simulink model "team_project_state_and_cds_adj_integration"  (R2023b)
settings: Solver=FixedStepAuto  StartTime=0.0  StopTime=inf  FixedStep=0.01  RelTol=1e-3  EnableMultiTasking=on
InitFcn:
  | params
  | pin_params
undefined symbols (not defined in the file or in its folder): b, den_Gd, encoder_scale, f, J, Kb, KD, Kf, KI, Km, KP, l, L, num_Gd, r, R, Vlim
libraries: arduinolib x17, arduinosensorlib x6, simulink x2
settings Model: SimulationMode=external  ExtModeTrigDuration=2  Creator=권주성  LastModifiedBy=SJ
settings SolverCC: AutoInsertRateTranBlk=on
settings OptimizationCC: EnhancedBackFolding=on  PassReuseOutputArgsAs=Individual arguments  ZeroExternalMemoryAtStartup=off  ZeroInternalMemoryAtStartup=off  MaxStackSize=64  OptimizeBlockOrder=speed  DifferentSizesBufferReuse=on  OptimizationCustomize=off  EfficientTunableParamExpr=on
settings DebuggingCC: ParameterPrecisionLossMsg=none  ParameterTunabilityLossMsg=error
settings HardwareCC: ProdBitPerInt=16  ProdBitPerPointer=16  ProdBitPerSizeT=16  ProdBitPerPtrDiffT=16  ProdLargestAtomicFloat=None  ProdWordSize=8  ProdHWDeviceType=Atmel->AVR
settings SFSimCC: MATLABDynamicMemAlloc=off
settings RTWCC: Description=Embedded Coder  SystemTargetFile=ert.tlc  HardwareBoard=Arduino Mega 2560  TemplateMakefile=ert_default_tmf  Toolchain=Arduino AVR  BuildConfiguration=Faster Runs
settings CodeAppCC: ForceParamTrailComments=on  IgnoreCustomStorageClasses=off  OperatorAnnotations=on  SimulinkDataObjDesc=on  SFDataObjDesc=on  InsertBlockDesc=on
settings ERTTargetCC: SupportContinuousTime=on  SupportVariableSizeSignals=on  ExtMode=on  ExtModeTransport=3  ExtModeStaticAlloc=on  ExtModeAutomaticAllocSize=off  ExtModeStaticAllocSize=2048  ExtModeMexFile=ext_xcp  ExtModeMexArgs=1 3 921600  ExtModeIntrfLevel=Level2 - Open

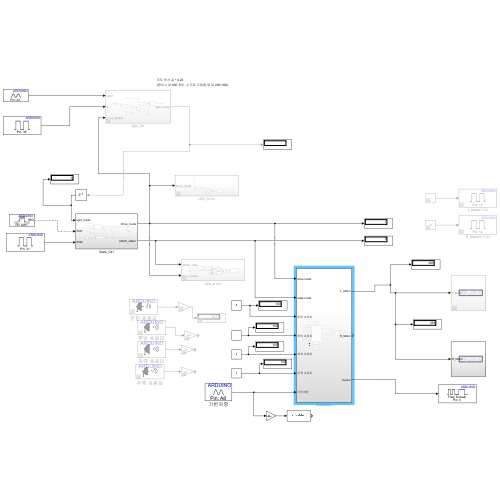
[thumbnail: Simulink's stored preview of the top-level diagram]
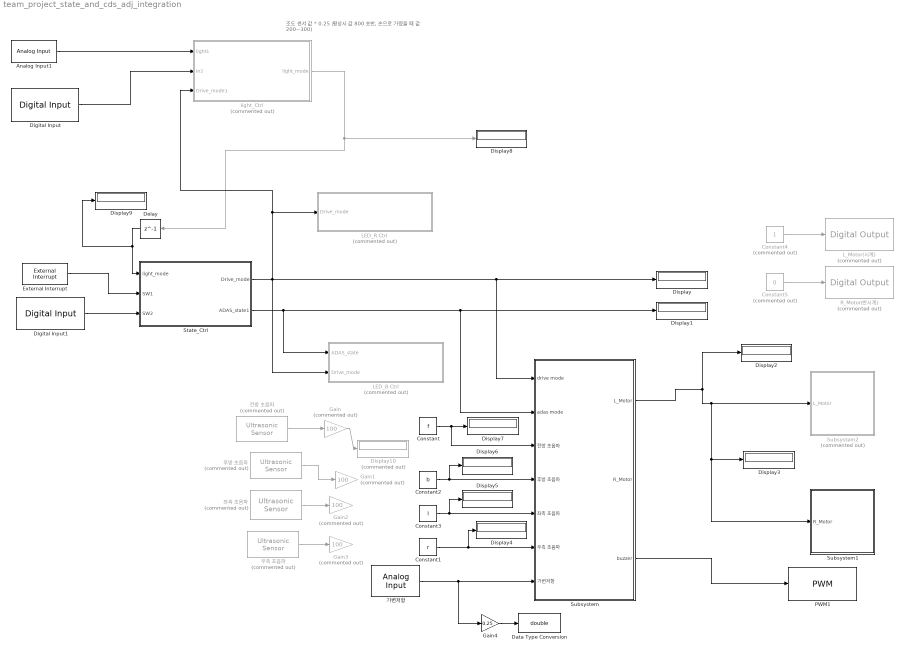
== system team_project_state_and_cds_adj_integration ==
  note: 조도 센서 값 * 0.25
      | (평상시 값 800 초반, 손으로 가렸을 때 값 200~300)
  Analog Input1 : arduinolib/Analog Input  pinNumber=BS  ReadResultsOnly=off  ConversionTriggerSource=Software  ExternalTriggerType=uint32( 0 )  OutputDataType=uint16  EnableConversionCompleteNotify=off  EnableOuputStatus=off  SampleTime=-1  blockPlatform=arduino
  Constant : Constant  Value=f
  Constant1 : Constant  Value=r
  Constant2 : Constant  Value=b
  Constant3 : Constant  Value=l
  Constant4 : Constant  Commented=on
  Constant5 : Constant  Commented=on  Value=0
  Data Type Conversion : DataTypeConversion  OutDataTypeStr=double  SaturateOnIntegerOverflow=off  RndMeth=Floor
  Delay : Delay  DelayLength=1
  Digital Input : arduinolib/Digital Input  pinNumber=SW3  mode=Default  Direction=input  SampleTime=0.1  blockPlatform=arduino
  Digital Input1 : arduinolib/Digital Input  pinNumber=SW2  mode=Default  Direction=input  SampleTime=0.1  blockPlatform=arduino
  Display{,1..9} (10 alike) : Display
  Display10 : Display  Commented=on
  External Interrupt : arduinolib/External Interrupt  Pin=SW1  PullUp=off  Mode=RISING  InterruptSimulationInput=off
  Gain{,1..3} (4 alike) : Gain  Commented=on  Gain=100
  Gain4 : Gain  Gain=0.25
  LED_B Ctrl : Subsystem  Commented=on
  LED_R Ctrl : Subsystem  Commented=on
  L_Motor(시계) : arduinolib/Digital Output  Commented=on  pinNumber=Motor_L_Direction  Direction=output  blockPlatform=arduino
  PWM1 : arduinolib/PWM  pinNumber=Buzzer  frequencyType=Default  desiredFrequency=490.2  achievableFrequency=490.2
  R_Motor(반시계) : arduinolib/Digital Output  Commented=on  pinNumber=Motor_R_Direction  Direction=output  blockPlatform=arduino
  State_Ctrl : Subsystem
  Subsystem : Subsystem
  Subsystem1 : Subsystem
  Subsystem2 : Subsystem  Commented=on
  light_Ctrl : Subsystem  Commented=on
  가변저항 : arduinolib/Analog Input  pinNumber=VR  ReadResultsOnly=off  ConversionTriggerSource=Software  ExternalTriggerType=uint32( 0 )  OutputDataType=uint16  EnableConversionCompleteNotify=off  EnableOuputStatus=off  SampleTime=-1  blockPlatform=arduino
  우측 초음파 : arduinosensorlib/Ultrasonic Sensor  Commented=on  NumSignalPins=2  TrigPin=R_Triger  EchoPin=R_Echo  SignalPin=3  SampleTime_=0.1  blockPlatform=ARDUINO
  전방 초음파 : arduinosensorlib/Ultrasonic Sensor  Commented=on  NumSignalPins=2  TrigPin=F_Triger  EchoPin=F_Echo  SignalPin=3  SampleTime_=0.1  blockPlatform=ARDUINO
  좌측 초음파 : arduinosensorlib/Ultrasonic Sensor  Commented=on  NumSignalPins=2  TrigPin=L_Triger  EchoPin=L_Echo  SignalPin=3  SampleTime_=0.1  blockPlatform=ARDUINO
  후방 초음파 : arduinosensorlib/Ultrasonic Sensor  Commented=on  NumSignalPins=2  TrigPin=B_Triger  EchoPin=B_Echo  SignalPin=3  SampleTime_=0.1  blockPlatform=ARDUINO
  wires:
  light_Ctrl/1(light_mode) -> Display8/1, Delay/1
  Analog Input1/1 -> light_Ctrl/1(light1)
  Delay/1 -> Display9/1, State_Ctrl/1(light_mode)
  State_Ctrl/2(ADAS_state1) -> LED_B Ctrl/1(ADAS_state), Subsystem/2(adas mode), Display1/1
  External Interrupt/1 -> State_Ctrl/2(SW1)
  State_Ctrl/1(Drive_mode) -> Subsystem/1(drive mode), Display/1, light_Ctrl/3(Drive_mode1), LED_R Ctrl/1(Drive_mode), LED_B Ctrl/2(Drive_mode)
  가변저항/1 -> Gain4/1, Subsystem/7(가변저항)
  Subsystem/3(buzzer) -> PWM1/1
  Constant3/1 -> Display5/1, Subsystem/5(좌측 초음파)
  Constant2/1 -> Display6/1, Subsystem/4(후방 초음파)
  좌측 초음파/1 -> Gain2/1
  전방 초음파/1 -> Gain/1
  Constant/1 -> Subsystem/3(전방 초음파), Display7/1
  우측 초음파/1 -> Gain3/1
  Constant1/1 -> Display4/1, Subsystem/6(우측 초음파)
  Subsystem/1(L_Motor) -> Display3/1, Subsystem1/1(R_Motor), Subsystem2/1(L_Motor), Display2/1
  후방 초음파/1 -> Gain1/1
  Digital Input1/1 -> State_Ctrl/3(SW2)
  Digital Input/1 -> light_Ctrl/2(In2)
  Constant4/1 -> L_Motor(시계)/1
  Constant5/1 -> R_Motor(반시계)/1
  Gain/1 -> Display10/1
  Gain4/1 -> Data Type Conversion/1

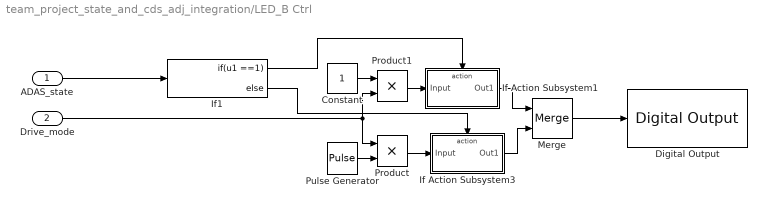
== system team_project_state_and_cds_adj_integration/LED_B Ctrl ==
  ADAS_state : Inport
  Drive_mode : Inport  Port=2
  Constant : Constant
  Digital Output : arduinolib/Digital Output  pinNumber=LED1_B  Direction=output  blockPlatform=arduino
  If Action Subsystem1 : Subsystem  TreatAsAtomicUnit=on
  If Action Subsystem3 : Subsystem  TreatAsAtomicUnit=on
  If1 : If  IfExpression=u1 ==1
  Merge : Merge
  Product : Product
  Product1 : Product
  Pulse Generator : DiscretePulseGenerator  PulseType=Time based  PulseWidth=50
  wires:
  If1/2 -> If Action Subsystem3/Action
  If Action Subsystem1/1(Out1) -> Merge/1
  ADAS_state/1 -> If1/1
  If1/1 -> If Action Subsystem1/Action
  Merge/1 -> Digital Output/1
  If Action Subsystem3/1(Out1) -> Merge/2
  Drive_mode/1 -> Product/1, Product1/2
  Pulse Generator/1 -> Product/2
  Constant/1 -> Product1/1
  Product1/1 -> If Action Subsystem1/1(Input)
  Product/1 -> If Action Subsystem3/1(Input)

== system team_project_state_and_cds_adj_integration/LED_R Ctrl ==
  Drive_mode : Inport
  Digital Output : arduinolib/Digital Output  pinNumber=LED1_R  Direction=output  blockPlatform=arduino
  If Action Subsystem1 : Subsystem  TreatAsAtomicUnit=on
  If Action Subsystem3 : Subsystem  TreatAsAtomicUnit=on
  If1 : If  IfExpression=u1 ==1
  Merge : Merge
  wires:
  If1/2 -> If Action Subsystem3/Action
  If Action Subsystem1/1(Out1) -> Merge/1
  Drive_mode/1 -> If1/1
  If1/1 -> If Action Subsystem1/Action
  Merge/1 -> Digital Output/1
  If Action Subsystem3/1(Out1) -> Merge/2

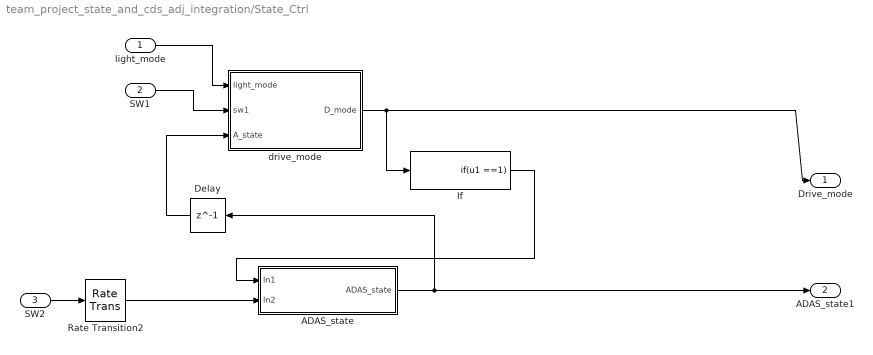
== system team_project_state_and_cds_adj_integration/State_Ctrl ==
  light_mode : Inport
  SW1 : Inport  Port=2
  SW2 : Inport  Port=3
  ADAS_state : Subsystem
  Delay : Delay  DelayLength=1
  If : If  IfExpression=u1 ==1  ShowElse=off
  Rate Transition2 : RateTransition  Integrity=off  OutPortSampleTime=0.2
  drive_mode : Subsystem
  Drive_mode : Outport
  ADAS_state1 : Outport  Port=2
  wires:
  If/1 -> ADAS_state/1(In1)
  drive_mode/1(D_mode) -> If/1, Drive_mode/1
  ADAS_state/1(ADAS_state) -> Delay/1, ADAS_state1/1
  SW1/1 -> drive_mode/2(sw1)
  Delay/1 -> drive_mode/3(A_state)
  light_mode/1 -> drive_mode/1(light_mode)
  SW2/1 -> Rate Transition2/1
  Rate Transition2/1 -> ADAS_state/2(In2)

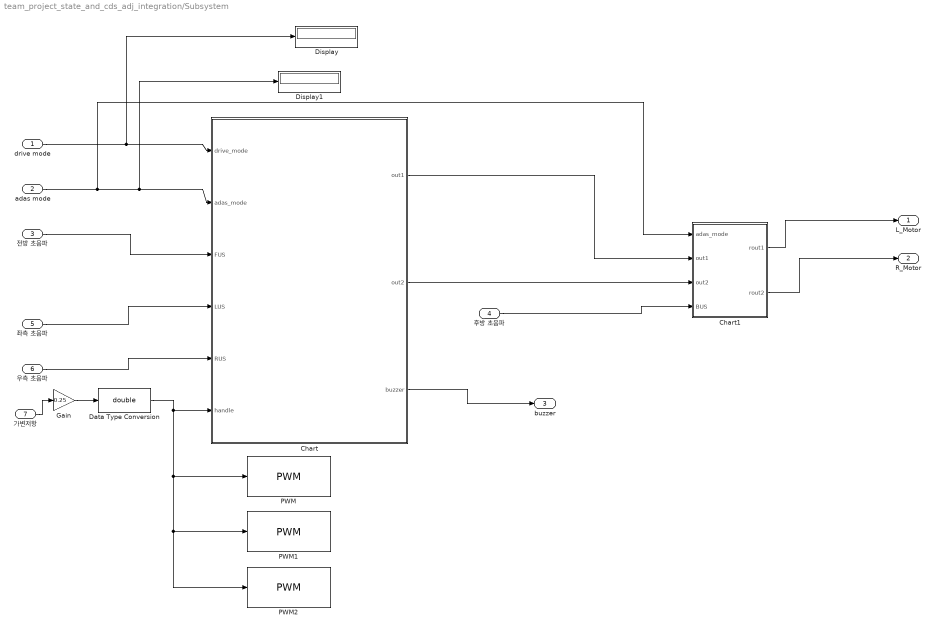
== system team_project_state_and_cds_adj_integration/Subsystem ==
  drive mode : Inport
  adas mode : Inport  Port=2
  전방 초음파 : Inport  Port=3
  후방 초음파 : Inport  Port=4
  좌측 초음파 : Inport  Port=5
  우측 초음파 : Inport  Port=6
  가변저항 : Inport  Port=7
  Chart : Stateflow chart  TreatAsAtomicUnit=on
  Chart1 : Stateflow chart  TreatAsAtomicUnit=on
  Data Type Conversion : DataTypeConversion  OutDataTypeStr=double  SaturateOnIntegerOverflow=off  RndMeth=Floor
  Display : Display
  Display1 : Display
  Gain : Gain  Gain=0.25
  PWM : arduinolib/PWM  pinNumber=RGB_LED_1  frequencyType=Default  desiredFrequency=490.2  achievableFrequency=490.2
  PWM1 : arduinolib/PWM  pinNumber=RGB_LED_2  frequencyType=Default  desiredFrequency=490.2  achievableFrequency=490.2
  PWM2 : arduinolib/PWM  pinNumber=RGB_LED_3  frequencyType=Default  desiredFrequency=490.2  achievableFrequency=490.2
  L_Motor : Outport
  R_Motor : Outport  Port=2
  buzzer : Outport  Port=3
  wires:
  drive mode/1 -> Chart/1(drive_mode), Display/1
  adas mode/1 -> Chart1/1(adas_mode), Chart/2(adas_mode), Display1/1
  전방 초음파/1 -> Chart/3(FUS)
  후방 초음파/1 -> Chart1/4(BUS)
  좌측 초음파/1 -> Chart/4(LUS)
  우측 초음파/1 -> Chart/5(RUS)
  Chart/3(buzzer) -> buzzer/1
  Chart/1(out1) -> Chart1/2(out1)
  Chart/2(out2) -> Chart1/3(out2)
  Chart1/1(rout1) -> L_Motor/1
  Chart1/2(rout2) -> R_Motor/1
  가변저항/1 -> Gain/1
  Gain/1 -> Data Type Conversion/1
  Data Type Conversion/1 -> PWM2/1, PWM1/1, PWM/1, Chart/6(handle)

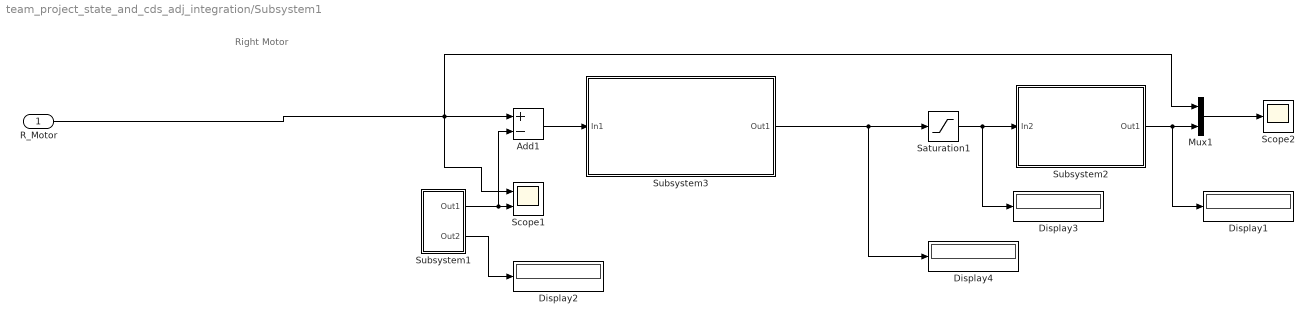
== system team_project_state_and_cds_adj_integration/Subsystem1 ==
  note: Right Motor
  R_Motor : Inport
  Add1 : Sum  Inputs=+-
  Display{1..4} (4 alike) : Display
  Mux1 : Mux  Inputs=2
  Saturation1 : Saturate  UpperLimit=12  LowerLimit=0
  Scope1 : Scope  NumInputPorts=2
  Scope2 : Scope
  Subsystem1 : Subsystem
  Subsystem2 : Subsystem
  Subsystem3 : Subsystem
  wires:
  Subsystem1/1(Out1) -> Add1/2, Scope1/2
  Subsystem3/1(Out1) -> Display4/1, Saturation1/1
  Saturation1/1 -> Subsystem2/1(In2), Display3/1
  Subsystem1/2(Out2) -> Display2/1
  Subsystem2/1(Out1) -> Display1/1, Mux1/2
  Mux1/1 -> Scope2/1
  Add1/1 -> Subsystem3/1(In1)
  R_Motor/1 -> Mux1/1, Scope1/1, Add1/1

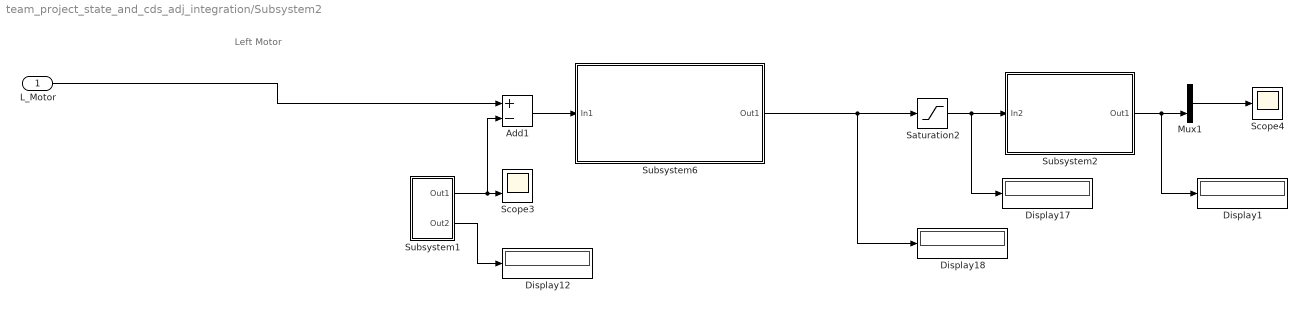
== system team_project_state_and_cds_adj_integration/Subsystem2 ==
  note: Left Motor
  L_Motor : Inport
  Add1 : Sum  Inputs=+-
  Display{1,12,17..18} (4 alike) : Display
  Mux1 : Mux  Inputs=2
  Saturation2 : Saturate  UpperLimit=12  LowerLimit=0
  Scope3 : Scope  NumInputPorts=2
  Scope4 : Scope
  Subsystem1 : Subsystem
  Subsystem2 : Subsystem
  Subsystem6 : Subsystem
  wires:
  Subsystem2/1(Out1) -> Display1/1, Mux1/2
  Subsystem1/2(Out2) -> Display12/1
  Subsystem6/1(Out1) -> Display18/1, Saturation2/1
  Add1/1 -> Subsystem6/1(In1)
  Mux1/1 -> Scope4/1
  Subsystem1/1(Out1) -> Add1/2, Scope3/2
  Saturation2/1 -> Subsystem2/1(In2), Display17/1
  L_Motor/1 -> Add1/1

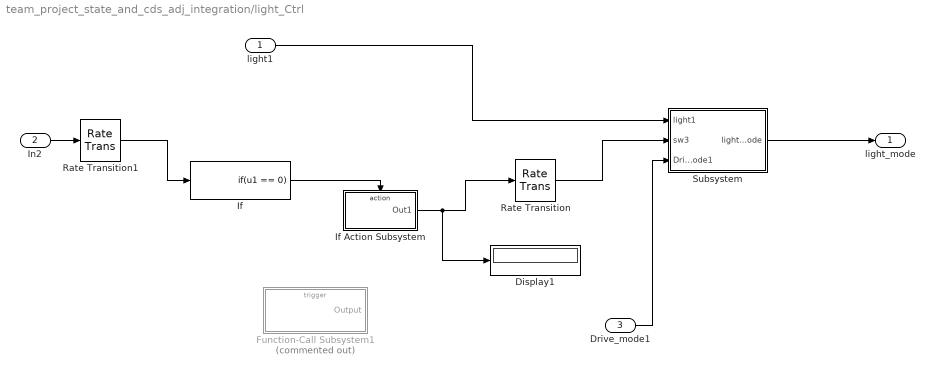
== system team_project_state_and_cds_adj_integration/light_Ctrl ==
  light1 : Inport
  In2 : Inport  Port=2
  Drive_mode1 : Inport  Port=3
  Display1 : Display
  Function-Call Subsystem1 : Subsystem  Commented=on  TreatAsAtomicUnit=on
  If : If  IfExpression=u1 == 0  ShowElse=off
  If Action Subsystem : Subsystem  TreatAsAtomicUnit=on
  Rate Transition : RateTransition  Integrity=off
  Rate Transition1 : RateTransition  Integrity=off  OutPortSampleTime=0.2
  Subsystem : Subsystem
  light_mode : Outport
  wires:
  If Action Subsystem/1(Out1) -> Display1/1, Rate Transition/1
  In2/1 -> Rate Transition1/1
  Rate Transition/1 -> Subsystem/2(sw3)
  Drive_mode1/1 -> Subsystem/3(Drive_mode1)
  light1/1 -> Subsystem/1(light1)
  Subsystem/1(light_mode) -> light_mode/1
  If/1 -> If Action Subsystem/Action
  Rate Transition1/1 -> If/1

== system team_project_state_and_cds_adj_integration/LED_B Ctrl/If Action Subsystem1 ==
  Input : Inport
  Action Port : ActionPort  ActionPortLabel=if(u1 ==1)
  Out1 : Outport
  wires:
  Input/1 -> Out1/1

== system team_project_state_and_cds_adj_integration/LED_B Ctrl/If Action Subsystem3 ==
  Input : Inport
  Action Port : ActionPort  ActionPortLabel=else
  Out1 : Outport
  wires:
  Input/1 -> Out1/1

== system team_project_state_and_cds_adj_integration/LED_R Ctrl/If Action Subsystem1 ==
  Action Port : ActionPort  ActionPortLabel=if(u1 ==1)
  Constant : Constant
  Out1 : Outport
  wires:
  Constant/1 -> Out1/1

== system team_project_state_and_cds_adj_integration/LED_R Ctrl/If Action Subsystem3 ==
  Action Port : ActionPort  ActionPortLabel=else
  Constant : Constant  Value=0
  Out1 : Outport
  wires:
  Constant/1 -> Out1/1

== system team_project_state_and_cds_adj_integration/State_Ctrl/ADAS_state ==
  In1 : Inport
  In2 : Inport  Port=2
  If : If  IfExpression=u1 == 0  ShowElse=off
  If Action Subsystem : Subsystem  TreatAsAtomicUnit=on
  If Action Subsystem1 : Subsystem  TreatAsAtomicUnit=on
  Rate Transition2 : RateTransition  Integrity=off  OutPortSampleTime=0.2
  SW2 : Subsystem  Commented=on
  ADAS_state : Outport
  wires:
  In1/1 -> If Action Subsystem/Action
  If Action Subsystem/1(ADAS_state) -> ADAS_state/1
  In2/1 -> Rate Transition2/1
  Rate Transition2/1 -> If/1
  If/1 -> If Action Subsystem1/Action
  If Action Subsystem1/1(sw2) -> If Action Subsystem/1(sw2)

== system team_project_state_and_cds_adj_integration/State_Ctrl/drive_mode ==
  light_mode : Inport
  sw1 : Inport  Port=2
  A_state : Inport  Port=3
  Chart : Stateflow chart  TreatAsAtomicUnit=on
  Rate Transition : RateTransition  Integrity=off
  SW1 : Subsystem
  D_mode : Outport
  wires:
  SW1/1(Output) -> Rate Transition/1
  Rate Transition/1 -> Chart/1(sw1)
  Chart/1(drive_mode) -> D_mode/1
  sw1/1 -> SW1/Trigger
  A_state/1 -> Chart/3(A_state)
  light_mode/1 -> Chart/2(light_mode)

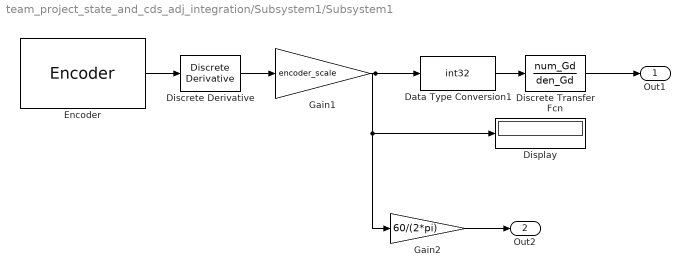
== system team_project_state_and_cds_adj_integration/Subsystem1/Subsystem1 ==
  Data Type Conversion1 : DataTypeConversion  OutDataTypeStr=int32  SaturateOnIntegerOverflow=off  RndMeth=Floor
  Discrete Transfer Fcn : DiscreteTransferFcn  Numerator=num_Gd  Denominator=den_Gd
  Discrete Derivative : simulink/Discrete/Discrete Derivative  gainval=1.0  ICPrevScaledInput=0.0  OutMin=[]  OutMax=[]  OutDataType=fixdt(1, 16)  OutScaling=2^-10  DoSatur=off
  Display : Display
  Encoder : arduinosensorlib/Encoder  InputA=20  InputB=21  Mode=No reset  SampleTime=-1
  Gain1 : Gain  Gain=encoder_scale
  Gain2 : Gain  Gain=60/(2*pi)
  Out1 : Outport
  Out2 : Outport  Port=2
  wires:
  Gain1/1 -> Display/1, Gain2/1, Data Type Conversion1/1
  Encoder/1 -> Discrete Derivative/1
  Gain2/1 -> Out2/1
  Data Type Conversion1/1 -> Discrete Transfer Fcn/1
  Discrete Derivative/1 -> Gain1/1
  Discrete Transfer Fcn/1 -> Out1/1

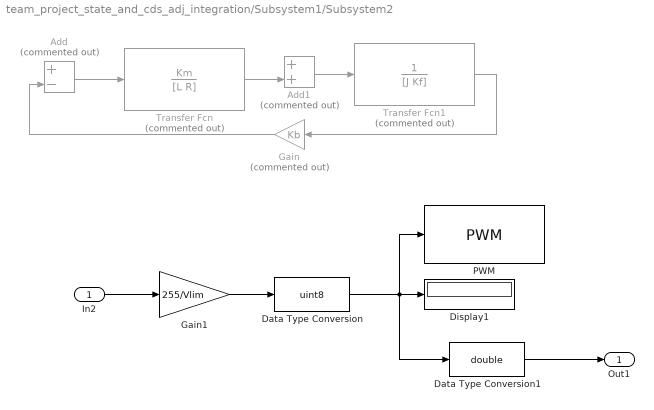
== system team_project_state_and_cds_adj_integration/Subsystem1/Subsystem2 ==
  In2 : Inport
  Add : Sum  Commented=on  Inputs=+-
  Add1 : Sum  Commented=on
  Data Type Conversion : DataTypeConversion  OutDataTypeStr=uint8  SaturateOnIntegerOverflow=off  RndMeth=Floor
  Data Type Conversion1 : DataTypeConversion  OutDataTypeStr=double  SaturateOnIntegerOverflow=off  RndMeth=Floor
  Display1 : Display
  Gain : Gain  Commented=on  Gain=Kb
  Gain1 : Gain  Gain=255/Vlim
  PWM : arduinolib/PWM  pinNumber=3  frequencyType=Default  desiredFrequency=490.2  achievableFrequency=490.2
  Transfer Fcn : TransferFcn  Commented=on  Numerator=Km  Denominator=[L R]
  Transfer Fcn1 : TransferFcn  Commented=on  Numerator=1  Denominator=[J Kf]
  Out1 : Outport
  wires:
  ? -> Add/1
  ? -> Add1/1
  Add/1 -> Transfer Fcn/1
  Add1/1 -> Transfer Fcn1/1
  Transfer Fcn/1 -> Add1/2
  Gain/1 -> Add/2
  Transfer Fcn1/1 -> Gain/1
  In2/1 -> Gain1/1
  Gain1/1 -> Data Type Conversion/1
  Data Type Conversion1/1 -> Out1/1
  Data Type Conversion/1 -> Data Type Conversion1/1, Display1/1, PWM/1

== system team_project_state_and_cds_adj_integration/Subsystem1/Subsystem3 ==
  In1 : Inport
  Derivative2 : Derivative  Commented=on
  Gain1 : Gain  Gain=KI
  Gain2 : Gain  Gain=KP
  Gain3 : Gain  Commented=on  Gain=KD
  Integrator2 : Integrator
  Subtract2 : Sum  Inputs=+++
  Out1 : Outport
  wires:
  Gain1/1 -> Integrator2/1
  Gain2/1 -> Subtract2/2
  Integrator2/1 -> Subtract2/1
  In1/1 -> Gain2/1, Gain3/1, Gain1/1
  Derivative2/1 -> Subtract2/3
  Gain3/1 -> Derivative2/1
  Subtract2/1 -> Out1/1

== system team_project_state_and_cds_adj_integration/Subsystem2/Subsystem1 ==
  Data Type Conversion1 : DataTypeConversion  OutDataTypeStr=int32  SaturateOnIntegerOverflow=off  RndMeth=Floor
  Discrete Transfer Fcn : DiscreteTransferFcn  Numerator=num_Gd  Denominator=den_Gd
  Discrete Derivative : simulink/Discrete/Discrete Derivative  gainval=1.0  ICPrevScaledInput=0.0  OutMin=[]  OutMax=[]  OutDataType=fixdt(1, 16)  OutScaling=2^-10  DoSatur=off
  Display : Display
  Encoder : arduinosensorlib/Encoder  InputA=18  InputB=19  Mode=No reset  SampleTime=-1
  Gain1 : Gain  Gain=encoder_scale
  Gain2 : Gain  Gain=60/(2*pi)
  Out1 : Outport
  Out2 : Outport  Port=2
  wires:
  Gain1/1 -> Display/1, Gain2/1, Data Type Conversion1/1
  Encoder/1 -> Discrete Derivative/1
  Gain2/1 -> Out2/1
  Data Type Conversion1/1 -> Discrete Transfer Fcn/1
  Discrete Derivative/1 -> Gain1/1
  Discrete Transfer Fcn/1 -> Out1/1

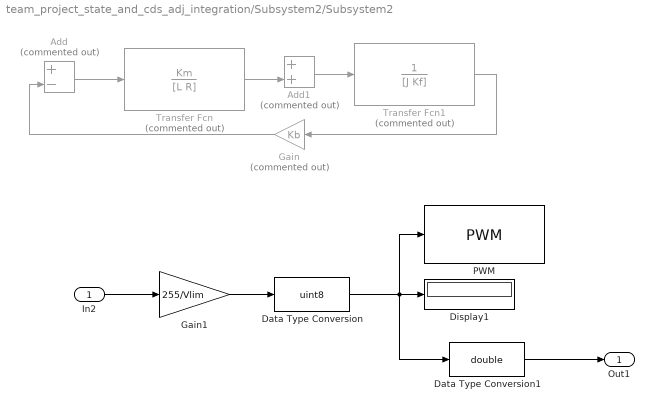
== system team_project_state_and_cds_adj_integration/Subsystem2/Subsystem2 ==
  In2 : Inport
  Add : Sum  Commented=on  Inputs=+-
  Add1 : Sum  Commented=on
  Data Type Conversion : DataTypeConversion  OutDataTypeStr=uint8  SaturateOnIntegerOverflow=off  RndMeth=Floor
  Data Type Conversion1 : DataTypeConversion  OutDataTypeStr=double  SaturateOnIntegerOverflow=off  RndMeth=Floor
  Display1 : Display
  Gain : Gain  Commented=on  Gain=Kb
  Gain1 : Gain  Gain=255/Vlim
  PWM : arduinolib/PWM  pinNumber=11  frequencyType=Default  desiredFrequency=490.2  achievableFrequency=490.2
  Transfer Fcn : TransferFcn  Commented=on  Numerator=Km  Denominator=[L R]
  Transfer Fcn1 : TransferFcn  Commented=on  Numerator=1  Denominator=[J Kf]
  Out1 : Outport
  wires:
  ? -> Add/1
  ? -> Add1/1
  Add/1 -> Transfer Fcn/1
  Add1/1 -> Transfer Fcn1/1
  Transfer Fcn/1 -> Add1/2
  Gain/1 -> Add/2
  Transfer Fcn1/1 -> Gain/1
  In2/1 -> Gain1/1
  Gain1/1 -> Data Type Conversion/1
  Data Type Conversion1/1 -> Out1/1
  Data Type Conversion/1 -> Data Type Conversion1/1, Display1/1, PWM/1

== system team_project_state_and_cds_adj_integration/Subsystem2/Subsystem6 ==
  In1 : Inport
  Derivative2 : Derivative
  Gain1 : Gain  Gain=KI
  Gain2 : Gain  Gain=KP
  Gain3 : Gain  Gain=KD
  Integrator2 : Integrator
  Subtract2 : Sum  Inputs=+++
  Out1 : Outport
  wires:
  Gain1/1 -> Integrator2/1
  Gain2/1 -> Subtract2/2
  Integrator2/1 -> Subtract2/1
  In1/1 -> Gain2/1, Gain3/1, Gain1/1
  Derivative2/1 -> Subtract2/3
  Gain3/1 -> Derivative2/1
  Subtract2/1 -> Out1/1

== system team_project_state_and_cds_adj_integration/light_Ctrl/Function-Call Subsystem1 ==
  function : TriggerPort  TriggerType=function-call  VariantControl=(inherit)
  Constant : Constant
  Constant1 : Constant  Value=3
  Delay : Delay  DelayLength=1
  Mod : Math  Operator=mod
  Sum : Sum  Inputs=|++
  Output : Outport
  wires:
  Constant/1 -> Sum/1
  Delay/1 -> Sum/2
  Constant1/1 -> Mod/2
  Sum/1 -> Delay/1, Mod/1
  Mod/1 -> Output/1

== system team_project_state_and_cds_adj_integration/light_Ctrl/If Action Subsystem ==
  Action Port : ActionPort  ActionPortLabel=if(u1 == 0)
  Constant : Constant
  Constant1 : Constant  Value=3
  Delay : Delay  DelayLength=1
  Mod : Math  Operator=mod
  Plus : Sum
  Out1 : Outport
  wires:
  Mod/1 -> Out1/1, Delay/1
  Constant/1 -> Plus/1
  Delay/1 -> Plus/2
  Plus/1 -> Mod/1
  Constant1/1 -> Mod/2

== system team_project_state_and_cds_adj_integration/light_Ctrl/Subsystem ==
  light1 : Inport
  sw3 : Inport  Port=2
  Drive_mode1 : Inport  Port=3
  Chart1 : Stateflow chart  TreatAsAtomicUnit=on
  Subsystem : Subsystem
  light_mode : Outport
  wires:
  Chart1/1(light_mode) -> Subsystem/2(light_mode), light_mode/1
  light1/1 -> Subsystem/1(light)
  sw3/1 -> Chart1/1(sw3)
  Drive_mode1/1 -> Chart1/2(Drive_mode)

== system team_project_state_and_cds_adj_integration/State_Ctrl/ADAS_state/If Action Subsystem ==
  sw2 : Inport
  Action Port : ActionPort  ActionPortLabel=if(u1 ==1)
  Chart : Stateflow chart  TreatAsAtomicUnit=on
  ADAS_state : Outport
  wires:
  sw2/1 -> Chart/1(sw2)
  Chart/1(ADAS_state) -> ADAS_state/1

== system team_project_state_and_cds_adj_integration/State_Ctrl/ADAS_state/If Action Subsystem1 ==
  Action Port : ActionPort  ActionPortLabel=if(u1 == 0)
  Constant2 : Constant
  Constant3 : Constant  Value=2
  Delay1 : Delay  DelayLength=1  InitialCondition=0
  Mod1 : Math  Operator=mod
  Sum : Sum  Inputs=|++
  sw2 : Outport
  wires:
  Mod1/1 -> sw2/1
  Delay1/1 -> Sum/2
  Constant3/1 -> Mod1/2
  Sum/1 -> Delay1/1, Mod1/1
  Constant2/1 -> Sum/1

== system team_project_state_and_cds_adj_integration/State_Ctrl/ADAS_state/SW2 ==
  function : TriggerPort  TriggerType=function-call  VariantControl=(inherit)
  Constant : Constant
  Constant1 : Constant  Value=2
  Delay : Delay  DelayLength=1  InitialCondition=0
  Mod : Math  Operator=mod
  Sum : Sum  Inputs=|++
  SW2 : Outport
  wires:
  Sum/1 -> Delay/1, Mod/1
  Constant1/1 -> Mod/2
  Mod/1 -> SW2/1
  Constant/1 -> Sum/1
  Delay/1 -> Sum/2

== system team_project_state_and_cds_adj_integration/State_Ctrl/drive_mode/SW1 ==
  function : TriggerPort  TriggerType=function-call  VariantControl=(inherit)
  Constant : Constant
  Constant1 : Constant  Value=2
  Delay : Delay  DelayLength=1
  Mod : Math  Operator=mod
  Sum : Sum  Inputs=|++
  Output : Outport
  wires:
  Constant/1 -> Sum/1
  Sum/1 -> Delay/1, Mod/1
  Constant1/1 -> Mod/2
  Delay/1 -> Sum/2
  Mod/1 -> Output/1

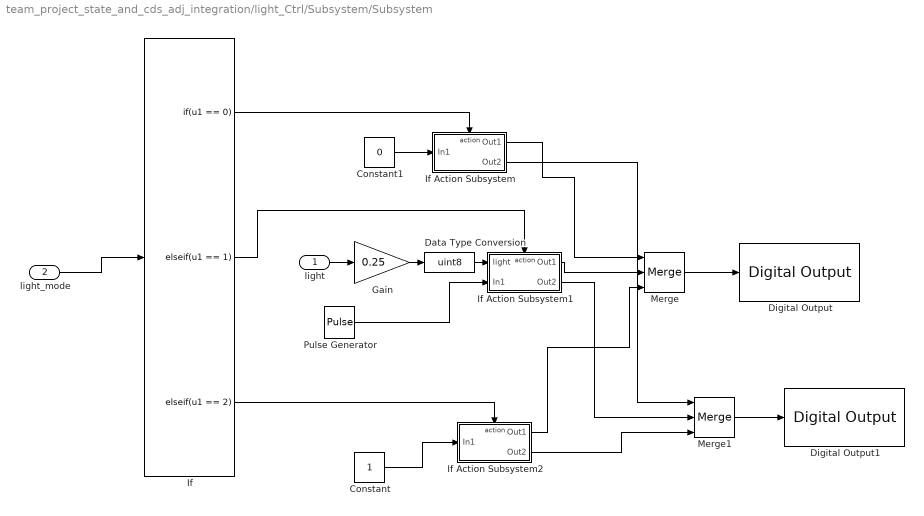
== system team_project_state_and_cds_adj_integration/light_Ctrl/Subsystem/Subsystem ==
  light : Inport
  light_mode : Inport  Port=2
  Constant : Constant
  Constant1 : Constant  Value=0
  Data Type Conversion : DataTypeConversion  OutDataTypeStr=uint8  SaturateOnIntegerOverflow=off  RndMeth=Floor
  Digital Output : arduinolib/Digital Output  pinNumber=LED2_R  Direction=output  blockPlatform=arduino
  Digital Output1 : arduinolib/Digital Output  pinNumber=LED2_B  Direction=output  blockPlatform=arduino
  Gain : Gain  Gain=0.25
  If : If  IfExpression=u1 == 0  ElseIfExpressions=u1 == 1, u1 == 2  ShowElse=off
  If Action Subsystem : Subsystem  TreatAsAtomicUnit=on
  If Action Subsystem1 : Subsystem  TreatAsAtomicUnit=on
  If Action Subsystem2 : Subsystem  TreatAsAtomicUnit=on
  Merge : Merge  Inputs=3
  Merge1 : Merge  Inputs=3
  Pulse Generator : DiscretePulseGenerator  PulseType=Time based  Period=0.2  PulseWidth=50
  wires:
  light_mode/1 -> If/1
  If/1 -> If Action Subsystem/Action
  If/2 -> If Action Subsystem1/Action
  If/3 -> If Action Subsystem2/Action
  Constant1/1 -> If Action Subsystem/1(In1)
  Constant/1 -> If Action Subsystem2/1(In1)
  If Action Subsystem/1(Out1) -> Merge/1
  If Action Subsystem1/1(Out1) -> Merge/2
  If Action Subsystem2/1(Out1) -> Merge/3
  Merge/1 -> Digital Output/1
  light/1 -> Gain/1
  Gain/1 -> Data Type Conversion/1
  Data Type Conversion/1 -> If Action Subsystem1/1(light)
  Pulse Generator/1 -> If Action Subsystem1/2(In1)
  If Action Subsystem1/2(Out2) -> Merge1/2
  If Action Subsystem/2(Out2) -> Merge1/1
  If Action Subsystem2/2(Out2) -> Merge1/3
  Merge1/1 -> Digital Output1/1

== system team_project_state_and_cds_adj_integration/light_Ctrl/Subsystem/Subsystem/If Action Subsystem ==
  In1 : Inport
  Action Port : ActionPort  ActionPortLabel=if(u1 == 0)
  Out1 : Outport
  Out2 : Outport  Port=2
  wires:
  In1/1 -> Out2/1, Out1/1

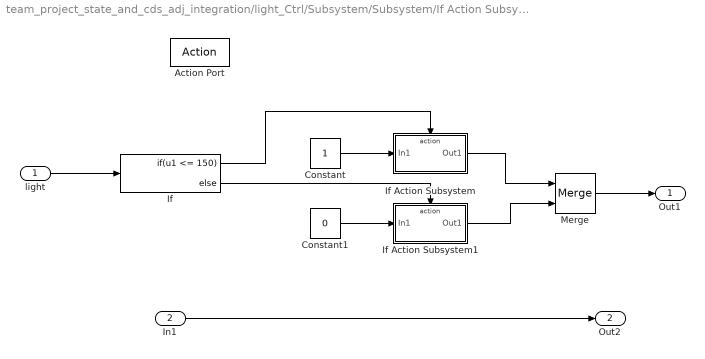
== system team_project_state_and_cds_adj_integration/light_Ctrl/Subsystem/Subsystem/If Action Subsystem1 ==
  light : Inport
  In1 : Inport  Port=2
  Action Port : ActionPort  ActionPortLabel=elseif(u1 == 1)
  Constant : Constant
  Constant1 : Constant  Value=0
  If : If  IfExpression=u1 <= 150
  If Action Subsystem : Subsystem  TreatAsAtomicUnit=on
  If Action Subsystem1 : Subsystem  TreatAsAtomicUnit=on
  Merge : Merge
  Out1 : Outport
  Out2 : Outport  Port=2
  wires:
  light/1 -> If/1
  Constant/1 -> If Action Subsystem/1(In1)
  Constant1/1 -> If Action Subsystem1/1(In1)
  If/1 -> If Action Subsystem/Action
  If/2 -> If Action Subsystem1/Action
  If Action Subsystem/1(Out1) -> Merge/1
  If Action Subsystem1/1(Out1) -> Merge/2
  Merge/1 -> Out1/1
  In1/1 -> Out2/1

== system team_project_state_and_cds_adj_integration/light_Ctrl/Subsystem/Subsystem/If Action Subsystem2 ==
  In1 : Inport
  Action Port : ActionPort  ActionPortLabel=elseif( u1 == 2)
  Out1 : Outport
  Out2 : Outport  Port=2
  wires:
  In1/1 -> Out2/1, Out1/1

== system team_project_state_and_cds_adj_integration/light_Ctrl/Subsystem/Subsystem/If Action Subsystem1/If Action Subsystem ==
  In1 : Inport
  Action Port : ActionPort  ActionPortLabel=if(u1 <= 150)
  Out1 : Outport
  wires:
  In1/1 -> Out1/1

== system team_project_state_and_cds_adj_integration/light_Ctrl/Subsystem/Subsystem/If Action Subsystem1/If Action Subsystem1 ==
  In1 : Inport
  Action Port : ActionPort  ActionPortLabel=else
  Out1 : Outport
  wires:
  In1/1 -> Out1/1

== stateflow chart team_project_state_and_cds_adj_integration/State_Ctrl/drive_mode/Chart ==
  state Drive_off
    en, du:
    drive_mode = 0;
    state_1 = sw1;
  state Drive_on
    en,du:
    drive_mode =1;
    state_1 = sw1;
    ADAS_state = A_state;
    Light_state = light_mode;
  (default) -> Drive_off
  Drive_off -> Drive_on : [state_1 ~= sw1]
  Drive_on -> Drive_off : [(state_1~=sw1) && (ADAS_state == 0) && (Light_state == 0)]
  data: sw1 input; light_mode input; state_1 local; drive_mode output; A_state input; ADAS_state local; Light_state local

== stateflow chart team_project_state_and_cds_adj_integration/light_Ctrl/Subsystem/Chart1 ==
  state light_auto
    en, du:
    light_mode = 1;
    state_1 = sw3;
  state light_off
    en, du:
    light_mode =0;
    state_1 = sw3;
  state light_on
    en,du:
    light_mode =2;
    state_1 = sw3;
  light_auto -> (junction 15) : [(state_1 ~= sw3) && (Drive_mode == 1)]
  (junction 12) -> light_auto
  (junction 15) -> light_on
  light_off -> (junction 12) : [(state_1 ~= sw3) && (Drive_mode == 1)]
  (default) -> light_off
  light_on -> light_off : [(state_1 ~= sw3) && (Drive_mode == 1)]
  data: sw3 input; Drive_mode input; state_1 local; light_mode output

== stateflow chart team_project_state_and_cds_adj_integration/Subsystem/Chart1 ==
  state adas_off
    en,du:
    rout1=out1;
    rout2=out2;
  state adas_on
    en,du:
    rout1=out1;
    rout2=out2;
  state adas_on_BUS
    en,du:
    rout1=out1*1.2;
    rout2=out2*1.2;
  adas_on_BUS -> adas_off [order 2] : [adas_mode==0]
  (default) -> adas_off
  adas_on -> adas_on_BUS [order 2] : [BUS<=10]
  adas_off -> adas_on : [adas_mode==1]
  adas_on -> adas_off [order 1] : [adas_mode==0]
  adas_on_BUS -> adas_on [order 1] : [BUS>10]
  data: adas_mode input; out1 input; out2 input; BUS input; rout1 output; rout2 output

== stateflow chart team_project_state_and_cds_adj_integration/State_Ctrl/ADAS_state/If Action Subsystem/Chart ==
  state adas_off
    en,du:
    ADAS_state = sw2;
    state_2 = sw2;
  state adas_on
    en,du:
    ADAS_state = sw2;
    state_2 =sw2;
  (default) -> adas_off
  adas_off -> adas_on : [state_2 ~= sw2]
  adas_on -> adas_off : [state_2 ~= sw2]
  data: sw2 input; state_2 local; ADAS_state output

== stateflow chart team_project_state_and_cds_adj_integration/Subsystem/Chart ==
  state drive_on_adas_on
    en, du:
    out1 = default;
    out2 = default;
  state drive_off
    en, du:
    out1 = 0;
    out2 = 0;
    steering = 0.02;
    default = 360;
  state drive_on_adas_off
    en, du:
    out1 = default*(1+(handle-128)/6.4/100);
    out2 = default*(1+(128-handle)/6.4/100);
    exit:
    buzzer = 0;
  state drive_on_adas_on_FUS
    en,du:
    out1 = 0;
    out2 = 0;
    buzzer = 1;
    exit:
    buzzer = 0;
  state drive_on_adas_on_LUS
    en,du:
    out1 = default*(1+(10-LUS)*steering);
    out2 = default*(1-(10-LUS)*steering);
  state drive_on_adas_on_RUS
    en,du:
    out1 = default*(1-(10-RUS)*steering);
    out2 = default*(1+(10-RUS)*steering);
  state drive_on_adas_on_LRUS
    en,du:
    out1 = default*(1-(LUS-RUS)*steering);
    out2 = default*(1+(LUS-RUS)*steering);
  drive_on_adas_on_FUS -> drive_on_adas_off [order 5] : [adas_mode ==0]
  (default) -> drive_off
  drive_on_adas_on -> drive_on_adas_on_FUS [order 2] : [FUS<=10]
  drive_on_adas_on_FUS -> drive_on_adas_on_LUS [order 4] : [LUS<=10&&FUS>10]
  drive_off -> drive_on_adas_off : [drive_mode==1]
  drive_on_adas_off -> drive_on_adas_on [order 2] : [adas_mode == 1]
  drive_on_adas_on_FUS -> drive_on_adas_on [order 1] : [LUS>10&&RUS>10&&FUS>10]
  drive_on_adas_off -> drive_off [order 1] : [drive_mode ==0]
  drive_on_adas_on_FUS -> drive_on_adas_on_LRUS [order 2] : [LUS<=10&&RUS<=10&&FUS>10]
  drive_on_adas_on -> drive_on_adas_off [order 1] : [adas_mode  == 0]
  drive_on_adas_on_RUS -> drive_on_adas_off [order 4] : [adas_mode ==0]
  drive_on_adas_on -> drive_on_adas_on_LUS [order 4] : [LUS<=10]
  drive_on_adas_on_LUS -> drive_on_adas_on [order 1] : [LUS>10]
  drive_on_adas_on -> drive_on_adas_on_RUS [order 3] : [RUS<=10]
  drive_on_adas_on_RUS -> drive_on_adas_on [order 1] : [RUS>10]
  drive_on_adas_on_LUS -> drive_on_adas_off [order 4] : [adas_mode ==0]
  drive_on_adas_on_LRUS -> drive_on_adas_off [order 4] : [adas_mode==0]
  drive_on_adas_on_LUS -> drive_on_adas_on_FUS [order 3] : [FUS<=10]
  drive_on_adas_on_LRUS -> drive_on_adas_on_FUS [order 1] : [FUS<=10]
  drive_on_adas_on_RUS -> drive_on_adas_on_FUS [order 2] : [FUS<=10]
  drive_on_adas_on_FUS -> drive_on_adas_on_RUS [order 3] : [RUS<=10&&FUS>10]
  drive_on_adas_on_RUS -> drive_on_adas_on_LRUS [order 3] : [LUS<=10]
  drive_on_adas_on_LRUS -> drive_on_adas_on_RUS [order 3] : [LUS>10]
  drive_on_adas_on_LUS -> drive_on_adas_on_LRUS [order 2] : [RUS<=10]
  drive_on_adas_on_LRUS -> drive_on_adas_on_LUS [order 2] : [RUS>10]
  data: drive_mode input; adas_mode input; FUS input; LUS input; RUS input; out1 output; out2 output; handle input double; buzzer output; steering local double; speed1 local double; speed2 local double; default local double
